simulink model "Pneumatic_act_PID"  (R2018b)
settings: Solver=ode15s  StartTime=0.0  StopTime=2  RelTol=5e-3
PreLoadFcn:
  | pneumaticInitialization
  | parametersMultibody
values from neighbouring files (symbols this model uses):
  base_breadth = 1    [parametersMultibody.m]
  base_height = 0.05    [parametersMultibody.m]
  base_length = 3.5    [parametersMultibody.m]
  box_breadth = 0.03    [parametersMultibody.m]
  box_height = 0.005    [parametersMultibody.m]
  box_height_s = 0.002    [parametersMultibody.m]
  box_length = 0.03    [parametersMultibody.m]
  box_yellow_breadth = 0.3    [parametersMultibody.m]
  box_yellow_height = 0.02    [parametersMultibody.m]
  box_yellow_length = 0.2    [parametersMultibody.m]
  frame_stand_breadth = 0.02    [parametersMultibody.m]
  frame_stand_height = 0.4280    (= 0.428)    [parametersMultibody.m]
  frame_stand_length = 0.02    [parametersMultibody.m]
undefined symbols (not defined in the file or in its folder): A_pipe, A_piston, delta_p, L_pipe, L_piston, p_init, sigbuilder_block, T_init, X, Y, Z
libraries: sm_lib x51, fl_lib x33, Contact_Forces_Lib x15, nesl_utility x7, simulink x2, Multibody_Parts_Lib x2, SimscapeFluids_lib x1, sm_backhoe_lib x1
(part 1 of 4)
settings Model: Creator=valakshe  LastModifiedBy=valakshe
settings SolverCC: MaxOrder=2  SolverJacobianMethodControl=SparsePerturbation  MinimalZcImpactIntegration=on
settings DataIOCC: ReturnWorkspaceOutputsName=tpc4ffeed1_4cd0_47cf_96e6_fe3975a5b339
settings OptimizationCC: EfficientMapNaN2IntZero=off
settings DebuggingCC: AlgebraicLoopMsg=none  ArtificialAlgebraicLoopMsg=none  MaxConsecutiveZCsMsg=none  MaskedZcDiagnostic=none  IgnoredZcDiagnostic=none  ModelReferenceExtraNoncontSigs=warning  SimStateInterfaceChecksumMismatchMsg=none  LibraryContextMissingDiagnostic=none
settings HardwareCC: TargetBitPerPointer=64  TargetBitPerSizeT=64  TargetBitPerPtrDiffT=64  TargetLongLongMode=on  TargetIntDivRoundTo=Zero  TargetEndianess=LittleEndian  TargetWordSize=64  TargetHWDeviceType=MATLAB Host  ProdEqTarget=off
settings SFSimCC: SimUseLocalCustomCode=off
settings CodeAppCC: MaxIdLength=128
settings GRTTargetCC: TargetLangStandard=C89/C90 (ANSI)  CombineOutputUpdateFcns=off  GRTInterface=on
settings DiagnosticsConfigSet: SimMechanicsRigidlyBoundBlock=none  SimMechanicsJointTargetOverSpecification=warning
settings ExplorerConfigSet: InternalSimMechanicsExplorerSettings="<ExplorerConfiguration><canonicalview>default</canonicalview><AnimationSetting><BasePlaybackSpeed>1.0</BasePlaybackSpeed><PlaybackSpeedFactor>0.25</PlaybackSpeedFactor></AnimationSetting><TilePanel><TileInfo><Tiles Columns=\"1\" Count=\"1\" Rows=\"1\"><Column Weight=\"1\"/><Row Weight=\"1\"/><Tile Height=\"1\" Width=\"1\" X=\"0\" Y=\"0\"/></Tiles></TileInfo><SceneInfo><SceneViewer><BGColor><R>1</R><G>1</G><B>1</B></BGColor><Camera><DoPerspective>off</DoPerspective><Position><X>2.26668765953207085</X><Y>-1.06668765756350892</Y><Z>0.816687631108211631</Z></Position><Center><X>1.19999996740823178</X><Y>3.45603302642771837e-08</Y><Z>-0.250000061015627661</Z></Center><Up><X>-0.408248290463863073</X><Y>0.408248290463863073</Y><Z>0.816496580927726145</Z></Up><ViewLimDist>1</ViewLimDist><YLim>1.08187340736389159</YLim><XLim>1.63872001409530643</XLim></Camera></SceneViewer></SceneInfo></TilePanel><MechEditorPanel><Cameras/><GfxPanelCameraMap/><VideoCreator><PlaybackSpeedRatio>1.0</PlaybackSpeedRatio><FrameRate>30</FrameRate><VideoFormat>Motion JPEG AVI</VideoFormat><FrameSize>auto</FrameSize></VideoCreator></MechEditorPanel></ExplorerConfiguration>"

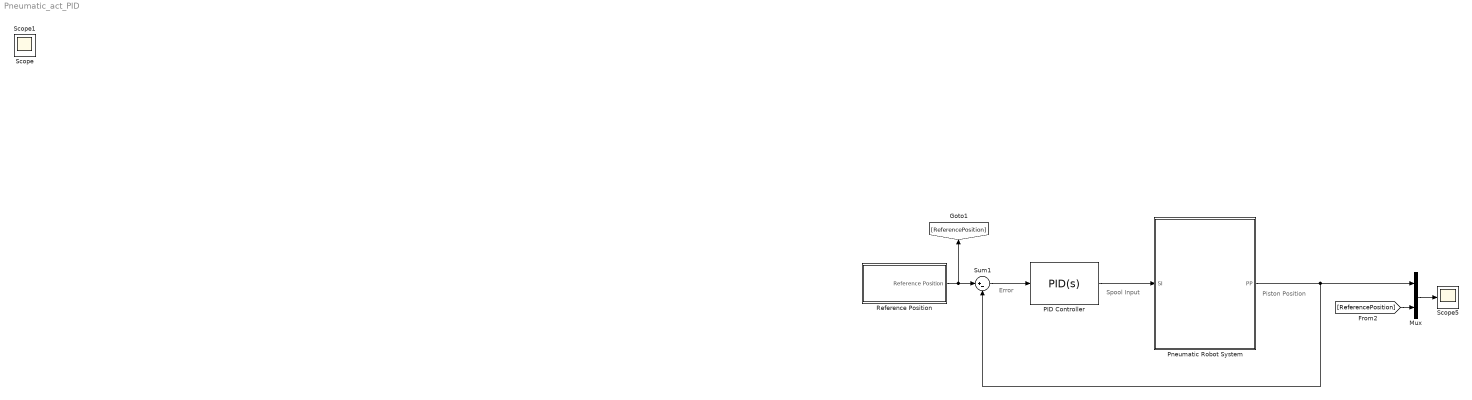
== system Pneumatic_act_PID ==
  note: Piston Position
  note: Spool Input
  note: Error
  Mux : Mux  Inputs=2
  "PID Controller " : simulink/Continuous/PID Controller  Controller=PID  Form=Parallel  TimeDomain=Continuous-time  SampleTime=-1  IntegratorMethod=Forward Euler  FilterMethod=Forward Euler  ControllerParametersSource=internal  P=10  I=15  D=0.075  UseFilter=on  N=250  TunerSelectOption=Transfer Function Based (PID Tuner App)  InitialConditionSource=internal  InitialConditionForIntegrator=0  InitialConditionForFilter=0  DifferentiatorICPrevScaledInput=0  ExternalReset=none  TrackingMode=off  Kt=1  LimitOutput=off  UpperSaturationLimit=2  LowerSaturationLimit=-2  LinearizeAsGain=on  AntiWindupMode=none  Kb=10  POutMin=[]  POutMax=[]  IOutMin=[]  IOutMax=[]  DOutMin=[]  DOutMax=[]  NOutMin=[]  NOutMax=[]  SumOutMin=[]  SumOutMax=[]  SaturationOutMin=[]  SaturationOutMax=[]  PParamMin=[]  PParamMax=[]  IParamMin=[]  IParamMax=[]  DParamMin=[]  DParamMax=[]  NParamMin=[]  NParamMax=[]  KbParamMin=[]  KbParamMax=[]  KtParamMin=[]  KtParamMax=[]  KbOutMin=[]  KbOutMax=[]  KtOutMin=[]  KtOutMax=[]  IntegratorOutMin=[]  IntegratorOutMax=[]  FilterOutMin=[]  FilterOutMax=[]  SumI1OutMin=[]  SumI1OutMax=[]  SumI2OutMin=[]  SumI2OutMax=[]  SumI3OutMin=[]  SumI3OutMax=[]  SumI4OutMin=[]  SumI4OutMax=[]  SumDOutMin=[]  SumDOutMax=[]  DifferentiatorOutMin=[]  DifferentiatorOutMax=[]  FilterDiffOutCoefMin=[]  FilterDiffOutCoefMax=[]  ReciprocalOutMin=[]  ReciprocalOutMax=[]  SumDenOutMin=[]  SumDenOutMax=[]  SumNumOutMin=[]  SumNumOutMax=[]  DivideOutMin=[]  DivideOutMax=[]  IntegratorContinuousStateAttributes=''  IntegratorStateMustResolveToSignalObject=off  IntegratorRTWStateStorageClass=Auto  FilterContinuousStateAttributes=''  FilterStateMustResolveToSignalObject=off  FilterRTWStateStorageClass=Auto  ParallelPVariant=InternalParameters  IdealPVariant=Disabled  IVariant=InternalParameters  DVariant=InternalParameters  IntegratorVariant=Continuous  SatVariant=Disabled  AWVariant=Passthrough  PCopyVariant=Disabled  TRVariant=Disabled  FdbkBlocksVariant=Forward  IdealPFdbkVariant=Disabled  SatFdbkVariant=Disabled  DerivativeFilterVariant=ContFilter  NVariant=InternalParameters  NCopyVariant=Disabled  FilterICVariant=InternalICsFilter  IntegratorICVariant=InternalICs  ExternalResetVariant=Disabled  TRSumVariant=Passthrough  SumFdbkVariant=Disabled  SumVariant=Sum_PID
  Pneumatic Robot System : Subsystem
      mask Display: image("Pneumatic Robot System.png")
  Reference Position : Subsystem  Tag=STV Subsys  LoadFcn=sigbuilder_block('load');  StartFcn=sigbuilder_block('start');  StopFcn=sigbuilder_block('stop');  ClipboardFcn=sigbuilder_block('clipboard');  mask(Sigbuilder block){tuvar=[0:10]}
      mask help: Simulink:masks:SigbuilderBlock_MD
      mask init:
      | if ~strcmp(get_param(bdroot(gcbh),'SimulationStatus'),'stopped') tuvar = sigbuilder_block('maskInit'); end
      settings: CopyFcn=sigbuilder_block('copy');  DeleteFcn=sigbuilder_block('delete');  ModelCloseFcn=sigbuilder_block('modelClose');  PreSaveFcn=sigbuilder_block('preSave');  PauseFcn=sigbuilder_block('pause');  ContinueFcn=sigbuilder_block('continue');  NameChangeFcn=sigbuilder_block('namechange');  OpenFcn=sigbuilder_block('open',[5.5 62 1429 778 ]);  CloseFcn=sigbuilder_block('close');
      mask Display: plot(0, 0, 100, 100,[2, 2, 32, 32, 2], [68, 8, 8, 68, 68],[32, 2], [38, 38], [32, 19, 2],[53, 60, 44], [32, 17, 17, 2],[16, 16, 31, 31]);txt = getActiveGroup(gcbh);text(2, 100, txt,'verticalAlignment', 'top');
  Scope5 : Scope
  Sum1 : Sum  Inputs=|+-
  Scope : Scope
  Scope1 : Scope
  wires:
  Mux/1 -> Scope5/1
  Reference Position/1(Reference Position) -> [ReferencePosition], Sum1/1
  Sum1/1 -> "PID Controller "/1
  [ReferencePosition] -> Mux/2
  "PID Controller "/1 -> Pneumatic Robot System/1(SI)
  Pneumatic Robot System/1(PP) -> Sum1/2, Mux/1

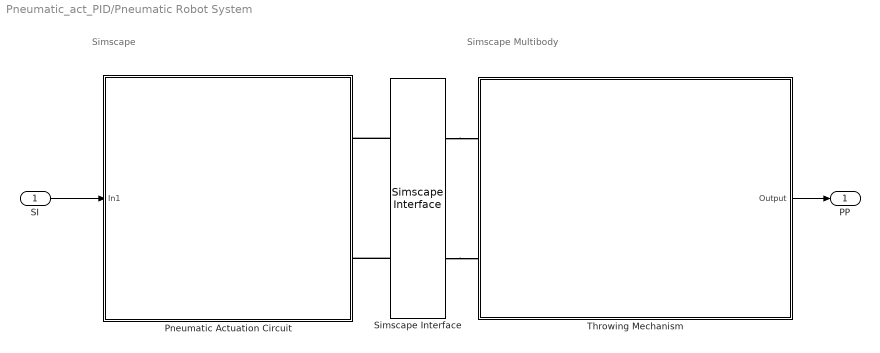
== system Pneumatic_act_PID/Pneumatic Robot System ==
  note: Simscape
  note: Simscape Multibody
  SI : Inport
  Pneumatic Actuation Circuit : Subsystem
  Simscape Interface : sm_backhoe_lib/Hydraulic Actuator/Simscape Interface  SystemSampleTime=-1
  Throwing Mechanism : Subsystem
      mask Display: image('Simscape_model.jpg')
  PP : Outport
  wires:
  SI/1 -> Pneumatic Actuation Circuit/1(In1)
  Throwing Mechanism/1(Output) -> PP/1
  connections:
  Simscape Interface/RConn1 -- Pneumatic Actuation Circuit/RConn1
  Simscape Interface/RConn2 -- Pneumatic Actuation Circuit/RConn2
  Simscape Interface/LConn1 -- Throwing Mechanism/LConn1
  Simscape Interface/LConn2 -- Throwing Mechanism/LConn2

== system Pneumatic_act_PID/Reference Position ==
  Demux : Demux  Tag=STV Demux  Outputs=1
  FromWs : FromWorkspace  Tag=STV FromWs  VariableName=tuvar  SampleTime=0
      SigBuilderData=|
      | common.afterFinalStr = 'Extrapolate'
      | common.sampleTime = '0'
      | dataSet.timeRange = [0 10]
      | dataSet.name = 'Group 1'
      | sbobj.Groups.Name = 'Group 1'
      | sbobj.Groups.Signals.Name = 'Reference Position'
      | sbobj.Groups.Signals.XData = [0 0.075 0.121 0.122 0.128 0.134 0.14 0.145 0.147 0.15 0.151 0.152 0.153 0.154 0.156 0.159 0.162 0.164 0.167 0.169 0.172 10]
      | sbobj.Groups.Signals.YData = [0 1.131e-06 1.364e-05 0.0002697 0.006792 0.02181 0.0413 0.04741 0.04823 0.04788 0.0475 0.0474 0.0473 0.04736 0.0477 0.0488 0.0508 0.05143 0.05177 0.05103 0.05108 0.05108]
  Reference Position : Outport  Tag=STV Outport
  wires:
  FromWs/1 -> Demux/1
  Demux/1 -> Reference Position/1
